simulink library "Math_Lib"  (R2016a)
settings: Solver=ode45  StartTime=0.0  StopTime=10.0  RelTol=1e-3
settings Model: Creator=sanny.omar  LastModifiedBy=Sanny
settings DataIOCC: LimitDataPoints=on  SaveFormat=Array
settings DebuggingCC: SolverPrmCheckMsg=warning
settings HardwareCC: ProdBitPerPointer=32  ProdLargestAtomicFloat=None  ProdIntDivRoundTo=Undefined  ProdEndianess=Unspecified  ProdWordSize=32  ProdHWDeviceType=32-bit Generic
settings ModelReferenceCC: PropagateSignalLabelsOutOfModel=off
settings ConfigComp: CovModelRefEnable=Off  CovSFcnEnable=off

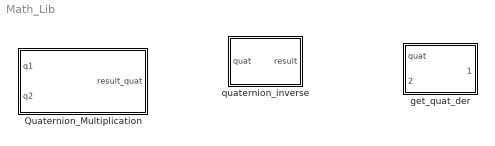
== system Math_Lib ==
  Quaternion_Multiplication : MATLAB Function  Description=Multiplies two quaternions  TreatAsAtomicUnit=on
  get_quat_der : MATLAB Function  TreatAsAtomicUnit=on
  quaternion_inverse : MATLAB Function  TreatAsAtomicUnit=on

== matlab function Math_Lib/quaternion_inverse ==
  data: quat input; result output
function result = quat_inv(quat)   
    size_q = size(quat)
    if(size_q(1) ~= 4 || size_q(2) ~= 1 || isreal(quat) == 0)
        a=5;
    end
    result = [quat(1); -quat(2:4)];

end

== matlab function Math_Lib/Quaternion_Multiplication ==
  data: q1 input; result_quat output; q2 input
% This function multiples two quaternions
function result_quat = quat_multiply(q1, q2)
    result_quat = zeros(4,1);
    mult_mat = [q1(1) -q1(2) -q1(3) -q1(4);
                q1(2)  q1(1) -q1(4)  q1(3);
                q1(3)  q1(4)  q1(1) -q1(2);
                q1(4) -q1(3)  q1(2)  q1(1);
                ];
            
    result_quat = mult_mat*q2;

== matlab function Math_Lib/get_quat_der ==
  data: quat input; quat_der output; ang_vel input
function quat_der = fcn(quat, ang_vel)
    ang_vel_quat = [ 0; ang_vel];
    quat_der = (1/2)*quat_multiply(ang_vel_quat, quat);
